simulink model "proc_control_ros2"  (R2024a)
settings: Solver=FixedStepAuto  StartTime=0.0  StopTime=inf  RelTol=1e-3
InitFcn:
  | InitProcControl;
StartFcn:
  | LoadParams;
values from neighbouring files (symbols this model uses):
  A = T200Spec16V{:,3}    [InitProcControl.m]
  dmax = simulation.drift.nominal .* rand(1,6)    [InitProcControl.m]
  dmin = -simulation.drift.nominal .* rand(1,6)    [InitProcControl.m]
  dSeedX = round(rand*10)    [InitProcControl.m]
  dts = 5    [InitProcControl.m]
  N = T200Spec16V{:,6}    [InitProcControl.m]
  PWM = T200Spec16V{:,1}    [InitProcControl.m]
  RPM = T200Spec16V{:,2}    [InitProcControl.m]
undefined symbols (not defined in the file or in its folder): angular_velocity, current_gains, data, data_SL_Info, DiscIntNeverNeededParam, elevation, heading, is_mpc_alive, is_trajectory_done, linear_acceleration, motor1, motor2, motor3, motor4, motor5, motor6, motor7, motor8, MPC, mpc_mode, mpc_status, orientation, physics, pose, position, simulation, simulink, target_reached, thrusters_status, thrusters_status_SL_Info, twist, x_vel_btm, y_vel_btm, z_vel_btm
libraries: ros2lib x79, aerolibutil x12, simulink x9, mpclib x3, embmathops x2, sharedtransform x2, robotcorelib x2, sharedTrackingLibrary x1
(part 1 of 3)
settings Model: SimulationMode=accelerator  PacingRate=1.400000  Creator=relat  LastModifiedBy=nimai
settings OptimizationCC: StrengthReduction=on  PassReuseOutputArgsAs=Individual arguments  ZeroExternalMemoryAtStartup=off  ZeroInternalMemoryAtStartup=off  EfficientFloat2IntCast=on  MaxStackSize=64  OptimizeBlockOrder=speed  MultiThreadedLoops=on  EfficientTunableParamExpr=on
settings DebuggingCC: ParameterTunabilityLossMsg=error
settings HardwareCC: ProdLargestAtomicInteger=Long  ProdLargestAtomicFloat=Double  ProdLongLongMode=on  ProdHWDeviceType=ARM Compatible->ARM 64-bit (LLP64)  TargetBitPerLong=64  TargetBitPerPointer=64  TargetBitPerSizeT=64  TargetBitPerPtrDiffT=64  TargetLargestAtomicFloat=Float  TargetIntDivRoundTo=Zero  TargetEndianess=LittleEndian  TargetWordSize=64  TargetHWDeviceType=AMD->x86-64 (Linux 64)
settings ModelReferenceCC: UpdateModelReferenceTargets=IfOutOfDate  EnableRefExpFcnMdlSchedulingChecks=on  EnableParallelModelReferenceBuilds=on
settings SFSimCC: SFSimEcho=off  MATLABDynamicMemAlloc=off  SimTargetLang=C++
settings RTWCC: Description=Embedded Coder  SystemTargetFile=ert.tlc  HardwareBoard=Robot Operating System 2 (ROS 2)  TLCOptions="-aInlineSetEventsForThisBaseRateFcn=TLC_FALSE -aSuppressMultiTaskScheduler=TLC_FALSE  -aRateBasedStepFcn=0"  GenCodeOnly=on  TemplateMakefile=ert_default_tmf  RetainRTWFile=on  Toolchain=Colcon Tools  BuildConfiguration=Faster Runs  TargetLang=C++
settings CodeAppCC: ForceParamTrailComments=on  IgnoreCustomStorageClasses=off  IgnoreTestpoints=on  OperatorAnnotations=on  SimulinkDataObjDesc=on  SFDataObjDesc=on  InsertBlockDesc=on
settings ERTTargetCC: TargetLangStandard=C++11 (ISO)  UtilityFuncGeneration=Shared location  CodeInterfacePackaging=C++ class  SupportVariableSizeSignals=on  RootIOFormat=Structure reference

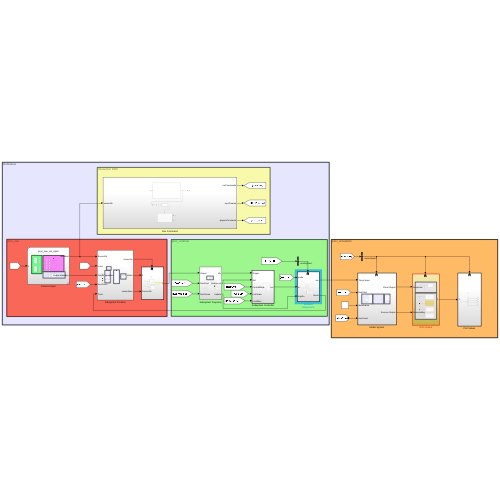
[thumbnail: Simulink's stored preview of the top-level diagram]
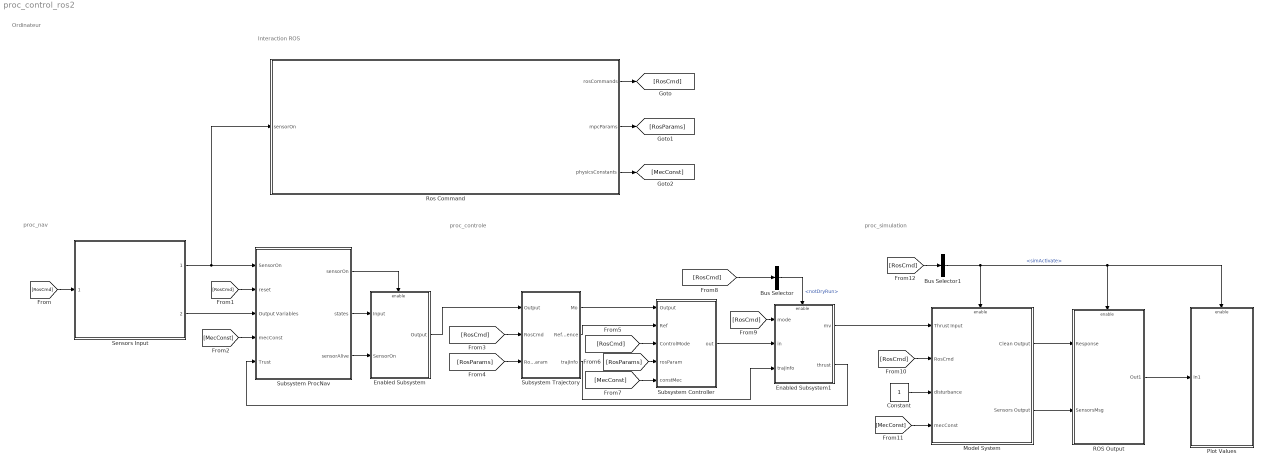
== system proc_control_ros2 ==
  note: Ordinateur
  note: proc_simulation
  note: proc_controle
  note: proc_nav
  note: Interaction ROS
  Bus Selector : BusSelector  OutputSignals=notDryRun
  Bus Selector1 : BusSelector  OutputSignals=simActivate
  Constant : Constant
  Enabled Subsystem : Subsystem  TreatAsAtomicUnit=on
  Enabled Subsystem1 : Subsystem  TreatAsAtomicUnit=on
  Model System : Subsystem  TreatAsAtomicUnit=on
  Plot Values : Subsystem  TreatAsAtomicUnit=on
  ROS Output : Subsystem  TreatAsAtomicUnit=on
  Ros Command : Subsystem
  Sensors Input : Subsystem  ReferencedSubsystem=proc_nav_ros_input
  Subsystem Controller : Subsystem  TreatAsAtomicUnit=on  SystemSampleTime=MPC.Ts
  Subsystem ProcNav : Subsystem
  Subsystem Trajectory : Subsystem
  wires:
  Ros Command/1(rosCommands) -> [RosCmd]
  Ros Command/2(mpcParams) -> [RosParams]
  Ros Command/3(physicsConstants) -> [MecConst]
  [RosCmd] -> Sensors Input/1
  Sensors Input/1 -> Ros Command/1(sensorOn), Subsystem ProcNav/1(SensorOn)
  [RosCmd] -> Subsystem ProcNav/2(reset)
  Sensors Input/2 -> Subsystem ProcNav/3(Output Variables)
  [MecConst] -> Subsystem ProcNav/4(mecConst)
  Subsystem ProcNav/1(sensorOn) -> Enabled Subsystem/Enable
  Subsystem ProcNav/2(states) -> Enabled Subsystem/1(Input)
  Subsystem ProcNav/3(sensorAlive) -> Enabled Subsystem/2(SensorOn)
  Enabled Subsystem/1(Output) -> Subsystem Trajectory/1(Output)
  [RosCmd] -> Subsystem Trajectory/2(RosCmd)
  [RosParams] -> Subsystem Trajectory/3(RosParam)
  Subsystem Trajectory/1(Mo) -> Subsystem Controller/1(Output)
  Subsystem Trajectory/2(Reference) -> Subsystem Controller/2(Ref)
  [RosCmd] -> Subsystem Controller/3(ControlMode)
  [RosParams] -> Subsystem Controller/4(rosParam)
  [MecConst] -> Subsystem Controller/5(constMec)
  Bus Selector/1 -> Enabled Subsystem1/Enable  "<notDryRun>"
  [RosCmd] -> Bus Selector/1
  [RosCmd] -> Enabled Subsystem1/1(mode)
  Subsystem Controller/1(out) -> Enabled Subsystem1/2(in)
  Subsystem Trajectory/3(trajInfo) -> Enabled Subsystem1/3(trajInfo)
  Enabled Subsystem1/2(thrust) -> Subsystem ProcNav/5(Trust)
  Enabled Subsystem1/1(mv) -> Model System/1(Thrust Input)
  [RosCmd] -> Model System/2(RosCmd)
  Constant/1 -> Model System/3(disturbance)
  [MecConst] -> Model System/4(mecConst)
  [RosCmd] -> Bus Selector1/1
  Bus Selector1/1 -> Plot Values/Enable, ROS Output/Enable, Model System/Enable  "<simActivate>"
  Model System/1(Clean Output) -> ROS Output/1(Response)
  Model System/2(Sensors Output) -> ROS Output/2(SensorsMsg)
  ROS Output/1(Out1) -> Plot Values/1(In1)

== system proc_control_ros2/Enabled Subsystem ==
  note: Skipped Commented Blocks
  Input : Inport
  SensorOn : Inport  Port=2
  Enable : EnablePort
  Send Sensor On : Subsystem
  Send auv states : Subsystem
  Output : Outport
  wires:
  Input/1 -> Output/1, Send auv states/1(Input)
  SensorOn/1 -> Send Sensor On/1(IsReached)

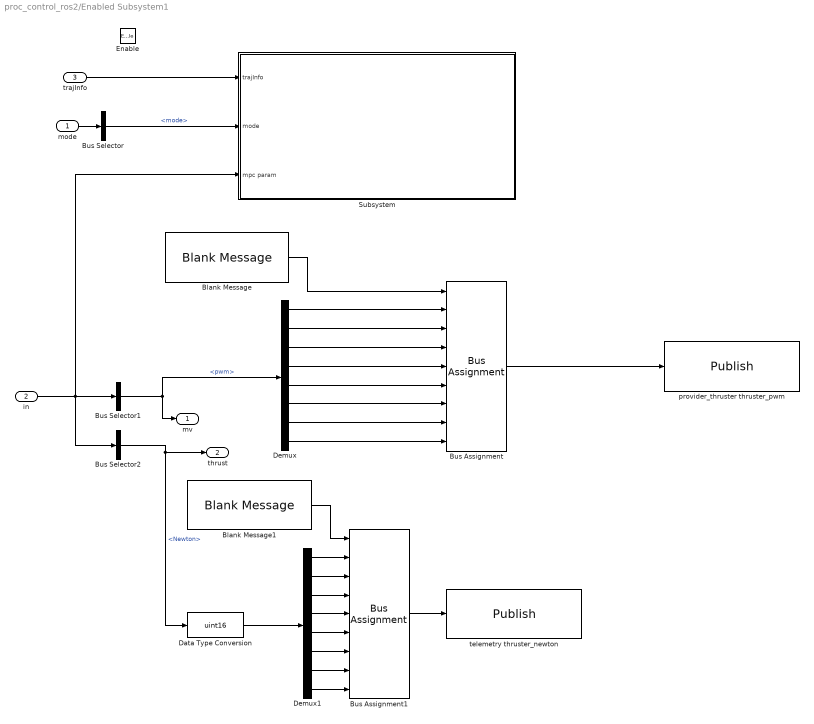
== system proc_control_ros2/Enabled Subsystem1 ==
  mode : Inport
  in : Inport  Port=2
  trajInfo : Inport  Port=3
  Enable : EnablePort
  Blank Message : ros2lib/Blank Message  messageClass=Message  entityType=sonia_common_ros2/MotorPwm  messageType=sonia_common_ros2/MotorPwm  SampleTime=inf
  Blank Message1 : ros2lib/Blank Message  messageClass=Message  entityType=sonia_common_ros2/MotorPwm  messageType=sonia_common_ros2/MotorPwm  SampleTime=inf
  Bus Assignment : BusAssignment  AssignedSignals=motor1,motor2,motor3,motor4,motor5,motor6,motor7,motor8
  Bus Assignment1 : BusAssignment  AssignedSignals=motor1,motor2,motor3,motor4,motor5,motor6,motor7,motor8
  Bus Selector : BusSelector  OutputSignals=mode
  Bus Selector1 : BusSelector  OutputSignals=pwm
  Bus Selector2 : BusSelector  OutputSignals=Newton
  Data Type Conversion : DataTypeConversion  OutDataTypeStr=uint16  SaturateOnIntegerOverflow=off  RndMeth=Floor
  Demux : Demux  Outputs=8
  Demux1 : Demux  Outputs=8
  Subsystem : Subsystem
  provider_thruster thruster_pwm : ros2lib/Publish  topicSource=Specify your own  topic=/provider_thruster/thruster_pwm  messageType=sonia_common_ros2/MotorPwm  QOSHistory=Keep last  QOSDepth=1  QOSReliability=Reliable  QOSDurability=Volatile  QOSDeadline=Inf  QOSLifespan=Inf  QOSLiveliness=Automatic  QOSLeaseDuration=Inf  QOSAvoidROSNamespaceConventions=off
  telemetry thruster_newton : ros2lib/Publish  topicSource=Specify your own  topic=/telemetry/thruster_newton  messageType=sonia_common_ros2/MotorPwm  QOSHistory=Keep last  QOSDepth=1  QOSReliability=Reliable  QOSDurability=Volatile  QOSDeadline=Inf  QOSLifespan=Inf  QOSLiveliness=Automatic  QOSLeaseDuration=Inf  QOSAvoidROSNamespaceConventions=off
  mv : Outport
  thrust : Outport  Port=2
  wires:
  trajInfo/1 -> Subsystem/1(trajInfo)
  mode/1 -> Bus Selector/1
  in/1 -> Subsystem/3(mpc param), Bus Selector2/1, Bus Selector1/1
  Bus Selector1/1 -> Demux/1, mv/1  "<pwm>"
  Bus Selector2/1 -> thrust/1, Data Type Conversion/1  "<Newton>"
  Blank Message/1 -> Bus Assignment/1
  Bus Assignment/1 -> provider_thruster thruster_pwm/1
  Bus Assignment1/1 -> telemetry thruster_newton/1
  Demux1/4 -> Bus Assignment1/5
  Demux1/1 -> Bus Assignment1/2
  Demux1/2 -> Bus Assignment1/3
  Blank Message1/1 -> Bus Assignment1/1
  Demux1/3 -> Bus Assignment1/4
  Demux1/5 -> Bus Assignment1/6
  Demux1/6 -> Bus Assignment1/7
  Demux1/7 -> Bus Assignment1/8
  Demux1/8 -> Bus Assignment1/9
  Data Type Conversion/1 -> Demux1/1
  Bus Selector/1 -> Subsystem/2(mode)  "<mode>"
  Demux/5 -> Bus Assignment/6
  Demux/6 -> Bus Assignment/7
  Demux/7 -> Bus Assignment/8
  Demux/8 -> Bus Assignment/9
  Demux/1 -> Bus Assignment/2
  Demux/2 -> Bus Assignment/3
  Demux/3 -> Bus Assignment/4
  Demux/4 -> Bus Assignment/5

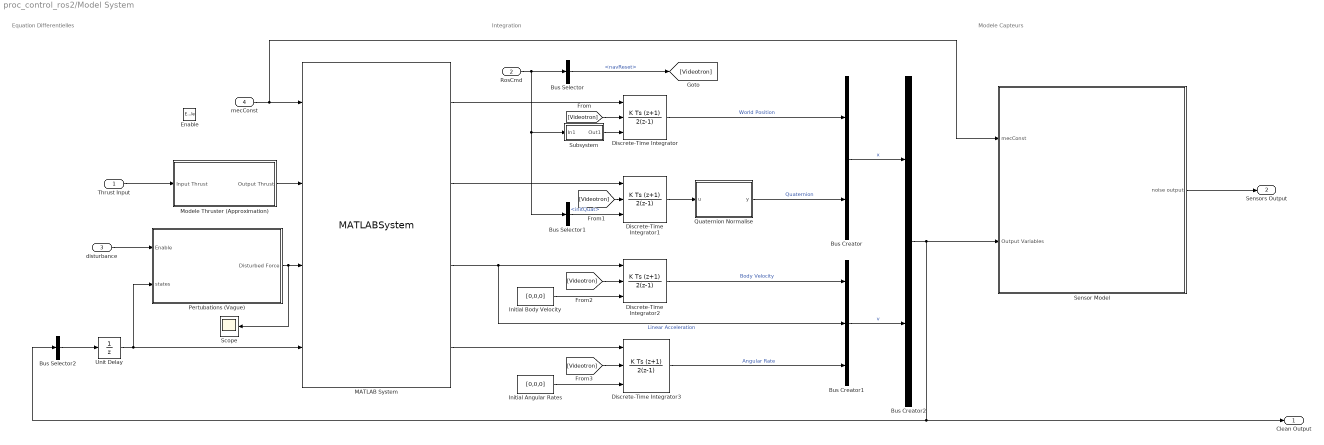
== system proc_control_ros2/Model System ==
  note: Modele Capteurs
  note: Integration
  note: Equation Differentielles
  Thrust Input : Inport
  RosCmd : Inport  Port=2
  disturbance : Inport  Port=3
  mecConst : Inport  Port=4
  Enable : EnablePort
  Bus Creator : BusCreator  Inputs=2
  Bus Creator1 : BusCreator  Inputs=3
  Bus Creator2 : BusCreator  Inputs=2
  Bus Selector : BusSelector  OutputSignals=navReset
  Bus Selector1 : BusSelector  OutputSignals=initQuat
  Bus Selector2 : BusSelector  OutputSignals=x.World Position,x.Quaternion,v.Body Velocity,v.Angular Rate  OutputAsBus=on
  Discrete-Time Integrator{,1..3} (4 alike) : DiscreteIntegrator  IntegratorMethod=Integration: Trapezoidal  ExternalReset=rising  InitialConditionSource=external  SampleTime=simulink.sampletime  ICPrevOutput=DiscIntNeverNeededParam  ICPrevScaledInput=DiscIntNeverNeededParam
  Initial Angular Rates : Constant  Value=[0,0,0]
  Initial Body Velocity : Constant  Value=[0,0,0]
  MATLAB System : MATLABSystem  System=AuvDifferentialEquation  simulation=simulation  MPC=MPC  useDynamicsConst=off  SimulateUsing=Code generation
      mask Type: AuvDifferentialEquation
      mask Display:
      | disp('AuvDifferentialEquation');
      | port_label('input',1,'mecConst');
      | port_label('input',2,'thrust');
      | port_label('input',3,'perturbations');
      | port_label('input',4,'states');
      | port_label('output',1,'Position_dot');
      | port_label('output',2,'Quaternion_dot');
      | port_label('output',3,'BodyVelocity_dot');
      | port_label('output',4,'AngularRates_dot');
  Modele Thruster (Approximation) : Subsystem
  Pertubations (Vague) : Subsystem
  Quaternion Normalise : MATLAB Function  TreatAsAtomicUnit=on
  Scope : Scope
  Sensor Model : Subsystem
  Subsystem : Subsystem
  Unit Delay : UnitDelay  InitialCondition=MPC.Xi  SampleTime=simulink.sampletime  HasFrameUpgradeWarning=on
  Clean Output : Outport
  Sensors Output : Outport  Port=2
  wires:
  Thrust Input/1 -> Modele Thruster (Approximation)/1(Input Thrust)
  disturbance/1 -> Pertubations (Vague)/1(Enable)
  Modele Thruster (Approximation)/1(Output Thrust) -> MATLAB System/2
  Pertubations (Vague)/1(Disturbed Force) -> Scope/1, MATLAB System/3
  mecConst/1 -> Sensor Model/1(mecConst), MATLAB System/1
  RosCmd/1 -> Bus Selector1/1, Subsystem/1(In1), Bus Selector/1
  Bus Selector/1 -> [Videotron]  "<navReset>"
  Subsystem/1(Out1) -> Discrete-Time Integrator/3
  [Videotron] -> Discrete-Time Integrator/2
  MATLAB System/1 -> Discrete-Time Integrator/1
  MATLAB System/2 -> Discrete-Time Integrator1/1
  Bus Selector1/1 -> Discrete-Time Integrator1/3  "<initQuat>"
  [Videotron] -> Discrete-Time Integrator1/2
  Discrete-Time Integrator1/1 -> Quaternion Normalise/1(u)
  [Videotron] -> Discrete-Time Integrator2/2
  Initial Body Velocity/1 -> Discrete-Time Integrator2/3
  Discrete-Time Integrator/1 -> Bus Creator/1  "World Position"
  Quaternion Normalise/1(y) -> Bus Creator/2  "Quaternion"
  MATLAB System/4 -> Discrete-Time Integrator3/1
  Initial Angular Rates/1 -> Discrete-Time Integrator3/3
  [Videotron] -> Discrete-Time Integrator3/2
  Discrete-Time Integrator2/1 -> Bus Creator1/1  "Body Velocity"
  Discrete-Time Integrator3/1 -> Bus Creator1/3  "Angular Rate"
  MATLAB System/3 -> Bus Creator1/2, Discrete-Time Integrator2/1  "Linear Acceleration"
  Bus Creator/1 -> Bus Creator2/1  "x"
  Bus Creator1/1 -> Bus Creator2/2  "v"
  Bus Creator2/1 -> Sensor Model/2(Output Variables), Bus Selector2/1, Clean Output/1
  Bus Selector2/1 -> Unit Delay/1
  Unit Delay/1 -> MATLAB System/4, Pertubations (Vague)/2(states)
  Sensor Model/1(noise output) -> Sensors Output/1

== system proc_control_ros2/Plot Values ==
  In1 : Inport
  Enable : EnablePort
  Bus Selector : BusSelector  OutputSignals=x.World Position,x.Quaternion,v.Body Velocity,v.Angular Rate
  Scope{,1..3} (4 alike) : Scope
  wires:
  In1/1 -> Bus Selector/1
  Bus Selector/1 -> Scope/1  "<World Position>"
  Bus Selector/2 -> Scope1/1  "<Quaternion>"
  Bus Selector/3 -> Scope2/1  "<Body Velocity>"
  Bus Selector/4 -> Scope3/1  "<Angular Rate>"

== system proc_control_ros2/ROS Output ==
  note: Sensor msg
  note: Simulator msg
  Response : Inport
  SensorsMsg : Inport  Port=2
  Enable : EnablePort
  Send DVL msg : Subsystem
  Send Depth msg : Subsystem
  Send IMU Msg : Subsystem
  Send Ping msg : Subsystem  Commented=on
  Send to Unity : Subsystem
  Out1 : Outport
  wires:
  Response/1 -> Send to Unity/1(Response), Out1/1
  SensorsMsg/1 -> Send Ping msg/1(Mesure), Send Depth msg/1(Mesure), Send DVL msg/1(Response), Send IMU Msg/1(Response)

== system proc_control_ros2/Ros Command ==
  sensorOn : Inport
  Bus Selector : BusSelector  OutputSignals=mode
  Get_ROS_param : Subsystem  TreatAsAtomicUnit=on
  If : If  IfExpression=u1 == 0  ShowElse=off
  Ros Command Manager : Subsystem
  Zero-Order Hold : ZeroOrderHold  SampleTime=simulink.ros.paramSampletime
  rosCommands : Outport
  mpcParams : Outport  Port=2
  physicsConstants : Outport  Port=3
  wires:
  Ros Command Manager/1(rosCommands) -> rosCommands/1, Bus Selector/1
  Get_ROS_param/1(mpcParams) -> mpcParams/1
  Zero-Order Hold/1 -> If/1
  Bus Selector/1 -> Zero-Order Hold/1  "<mode>"
  If/1 -> Get_ROS_param/Action
  sensorOn/1 -> Ros Command Manager/1(sensorOn)
  Get_ROS_param/2(physicsConstants) -> physicsConstants/1

== system proc_control_ros2/Subsystem Controller ==
  Output : Inport
  Ref : Inport  Port=2
  ControlMode : Inport  Port=3
  rosParam : Inport  Port=4
  constMec : Inport  Port=5
  Bus Selector : BusSelector  OutputSignals=mode
  Bus Selector1 : BusSelector  OutputSignals=current
  Controller List : Subsystem
  Delay : Delay  DelayLength=1  InitialCondition=zeros(1,8)  SampleTime=MPC.Ts
  If : If  IfExpression=u1 >= 0  ShowElse=off
  If Action Subsystem : Subsystem  TreatAsAtomicUnit=on
  Post Traitement : Subsystem
  out : Outport
  wires:
  Output/1 -> Controller List/1(mo), If Action Subsystem/2(mo)
  ControlMode/1 -> Bus Selector/1
  Bus Selector/1 -> Controller List/2(ControlMode), If Action Subsystem/1(mode), If/1  "<mode>"
  If/1 -> If Action Subsystem/Action
  rosParam/1 -> If Action Subsystem/4(mpcParams)
  If Action Subsystem/1(MPC param) -> Post Traitement/2(MpcParams), Controller List/4(mpc param)
  constMec/1 -> Controller List/5(constMec)
  Ref/1 -> Controller List/3(Ref)
  Controller List/1(Out1) -> Post Traitement/1(In1)
  Post Traitement/1(out) -> Bus Selector1/1, out/1
  Bus Selector1/1 -> Delay/1  "<current>"
  Delay/1 -> If Action Subsystem/3(Current)

== system proc_control_ros2/Subsystem ProcNav ==
  note: Skipped Commented Block
  note: Mettre les données
      | dans un bus
  note: Filtre EKF
  note: Pre traitement des mesures
  note: Conditions pour activer le kalman
  SensorOn : Inport
  reset : Inport  Port=2
  Output Variables : Inport  Port=3
  mecConst : Inport  Port=4
  Trust : Inport  Port=5
  AHRS/Detph Mesurments : Subsystem
  Bus Selector : BusSelector  OutputSignals=navReset
  Bus Selector1 : BusSelector  OutputSignals=NewDvlMsg
  Bus Selector2 : BusSelector  OutputSignals=new Pressure Msg
  DVL Measurements : Subsystem  TreatAsAtomicUnit=on
  Depth Measurements : Subsystem  TreatAsAtomicUnit=on
  Enabled Subsystem : Subsystem  TreatAsAtomicUnit=on
  Reset Logic : Subsystem
  State function arguments : Subsystem
  mux2Bus : Subsystem
  sensorOn : Outport
  states : Outport  Port=2
  sensorAlive : Outport  Port=3
  wires:
  reset/1 -> Bus Selector/1
  Bus Selector/1 -> Reset Logic/1(In1)  "<navReset>"
  SensorOn/1 -> sensorAlive/1, Reset Logic/2(2)
  Reset Logic/1(Out1) -> Enabled Subsystem/Enable, sensorOn/1
  Trust/1 -> State function arguments/1(thrust)
  mecConst/1 -> DVL Measurements/2(mecConst), Enabled Subsystem/5(mecConst), Depth Measurements/2(mecConst), State function arguments/2(mecConst)
  Output Variables/1 -> DVL Measurements/1(DVL Velocity), Bus Selector2/1, Depth Measurements/1(y), Bus Selector1/1, AHRS/Detph Mesurments/1(y)
  Bus Selector1/1 -> DVL Measurements/Enable  "<NewDvlMsg>"
  Bus Selector2/1 -> Depth Measurements/Enable  "<new Pressure Msg>"
  AHRS/Detph Mesurments/1(IMU) -> Depth Measurements/3(xhat), Enabled Subsystem/2(AHRS Mesurments)
  State function arguments/1(stateFuncArguments) -> Enabled Subsystem/1(stateFuncArguments)
  DVL Measurements/1(DVL Measurements) -> Enabled Subsystem/3("DVL Measurements ")
  Depth Measurements/1(Depth Measurements) -> Enabled Subsystem/4(Depth Measurements)
  Enabled Subsystem/1(xhat) -> mux2Bus/1(xhat)
  mux2Bus/1(states) -> states/1  "md"

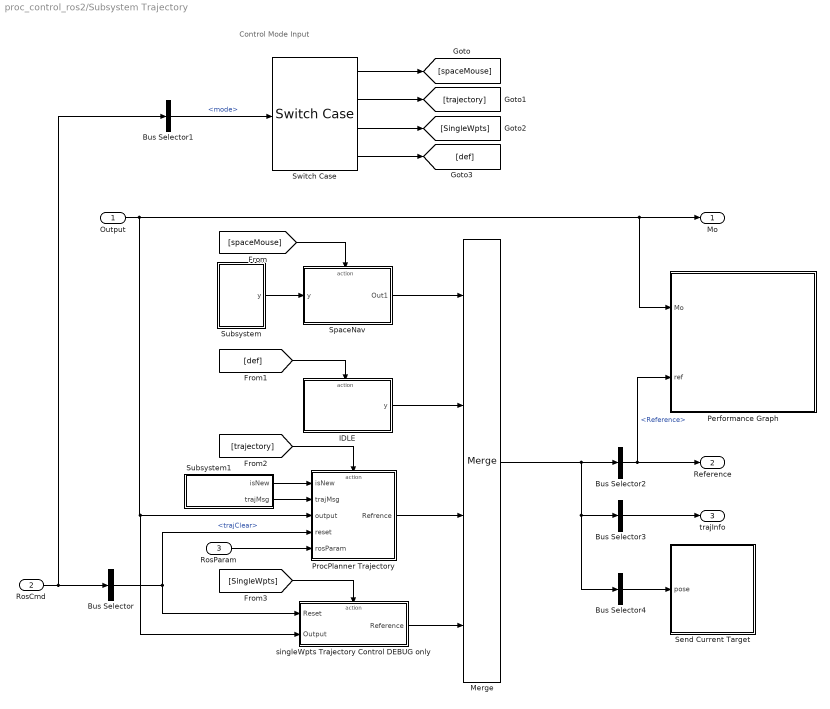
== system proc_control_ros2/Subsystem Trajectory ==
  note: Control Mode Input
  Output : Inport
  RosCmd : Inport  Port=2
  RosParam : Inport  Port=3
  Bus Selector : BusSelector  OutputSignals=trajClear
  Bus Selector1 : BusSelector  OutputSignals=mode
  Bus Selector2 : BusSelector  OutputSignals=Reference
  Bus Selector3 : BusSelector  OutputSignals=isReached,isTrajDone  OutputAsBus=on
  Bus Selector4 : BusSelector  OutputSignals=target  OutputAsBus=on
  IDLE : Subsystem  TreatAsAtomicUnit=on
  Merge : Merge  Inputs=4
  Performance Graph : Subsystem
  ProcPlanner Trajectory : Subsystem  TreatAsAtomicUnit=on
  Send Current Target : Subsystem
  SpaceNav : Subsystem  TreatAsAtomicUnit=on
  Subsystem : Subsystem
  Subsystem1 : Subsystem
  Switch Case : SwitchCase  CaseConditions={mode.traj.SpaceMouseMode,mode.traj.trajMode, mode.traj.singleWpts,}
  singleWpts Trajectory Control DEBUG only : Subsystem  TreatAsAtomicUnit=on
  Mo : Outport
  Reference : Outport  Port=2
  trajInfo : Outport  Port=3
  wires:
  RosCmd/1 -> Bus Selector1/1, Bus Selector/1
  Bus Selector1/1 -> Switch Case/1  "<mode>"
  Switch Case/1 -> [spaceMouse]
  Switch Case/2 -> [trajectory]
  Switch Case/3 -> [SingleWpts]
  Switch Case/4 -> [def]
  Output/1 -> singleWpts Trajectory Control DEBUG only/2(Output), ProcPlanner Trajectory/3(output), Performance Graph/1(Mo), Mo/1
  [spaceMouse] -> SpaceNav/Action
  Subsystem/1(y) -> SpaceNav/1(y)
  [def] -> IDLE/Action
  [trajectory] -> ProcPlanner Trajectory/Action
  Subsystem1/1(isNew) -> ProcPlanner Trajectory/1(isNew)
  Subsystem1/2(trajMsg) -> ProcPlanner Trajectory/2(trajMsg)
  Bus Selector/1 -> singleWpts Trajectory Control DEBUG only/1(Reset), ProcPlanner Trajectory/4(reset)  "<trajClear>"
  RosParam/1 -> ProcPlanner Trajectory/5(rosParam)
  [SingleWpts] -> singleWpts Trajectory Control DEBUG only/Action
  SpaceNav/1(Out1) -> Merge/1
  IDLE/1(y) -> Merge/2
  ProcPlanner Trajectory/1(Refrence) -> Merge/3
  singleWpts Trajectory Control DEBUG only/1(Reference) -> Merge/4
  Merge/1 -> Bus Selector4/1, Bus Selector3/1, Bus Selector2/1
  Bus Selector2/1 -> Performance Graph/2(ref), Reference/1  "<Reference>"
  Bus Selector3/1 -> trajInfo/1
  Bus Selector4/1 -> Send Current Target/1(pose)

== system proc_control_ros2/Enabled Subsystem/Send Sensor On ==
  IsReached : Inport
  Blank Message : ros2lib/Blank Message  messageClass=Message  entityType=std_msgs/Bool  messageType=std_msgs/Bool  SampleTime=inf
  Bus Assignment : BusAssignment  AssignedSignals=data
  Data Type Conversion : DataTypeConversion  OutDataTypeStr=boolean  SaturateOnIntegerOverflow=off  RndMeth=Floor
  Zero-Order Hold : ZeroOrderHold
  proc_control sensor_on : ros2lib/Publish  topicSource=Specify your own  topic=/proc_control/sensor_on  messageType=std_msgs/Bool  QOSHistory=Keep last  QOSDepth=1  QOSReliability=Reliable  QOSDurability=Volatile  QOSDeadline=Inf  QOSLifespan=Inf  QOSLiveliness=Automatic  QOSLeaseDuration=Inf  QOSAvoidROSNamespaceConventions=off
  wires:
  Bus Assignment/1 -> Zero-Order Hold/1
  Zero-Order Hold/1 -> proc_control sensor_on/1
  Data Type Conversion/1 -> Bus Assignment/2
  Blank Message/1 -> Bus Assignment/1
  IsReached/1 -> Data Type Conversion/1

== system proc_control_ros2/Enabled Subsystem/Send auv states ==
  Input : Inport
  Blank Message : ros2lib/Blank Message  messageClass=Message  entityType=nav_msgs/Odometry  messageType=nav_msgs/Odometry  SampleTime=inf
  Bus Assignment : BusAssignment  AssignedSignals=pose.pose.position.x,pose.pose.position.y,pose.pose.position.z,pose.pose.orientation.w,pose.pose.orientation.x,pose.pose.orientation.y,pose.pose.orientation.z,twist.twist.linear.x,twist.twist.linear.y,twist.twist.linear.z,twist.twist.angular.x,twist.twist.angular.y,twist.twist.angular.z
  Demux : Demux  Outputs=13
  Header Assignment : ros2lib/Header Assignment  SetFrameID=on  FrameID=NED  InsertTimeStamp=on  SetHeaderFieldName=Use the default header field name  HeaderFieldName=header
  bus2mux : Subsystem
  proc_nav auv_states : ros2lib/Publish  topicSource=Specify your own  topic=/proc_nav/auv_states  messageType=nav_msgs/Odometry  QOSHistory=Keep last  QOSDepth=1  QOSReliability=Reliable  QOSDurability=Volatile  QOSDeadline=Inf  QOSLifespan=5  QOSLiveliness=Automatic  QOSLeaseDuration=5  QOSAvoidROSNamespaceConventions=off
  wires:
  Blank Message/1 -> Header Assignment/1
  Input/1 -> bus2mux/1(Input)
  Header Assignment/1 -> Bus Assignment/1
  bus2mux/1(states) -> Demux/1
  Demux/1 -> Bus Assignment/2
  Demux/2 -> Bus Assignment/3
  Demux/3 -> Bus Assignment/4
  Demux/4 -> Bus Assignment/5
  Demux/5 -> Bus Assignment/6
  Demux/6 -> Bus Assignment/7
  Demux/7 -> Bus Assignment/8
  Demux/8 -> Bus Assignment/9
  Demux/9 -> Bus Assignment/10
  Demux/10 -> Bus Assignment/11
  Demux/11 -> Bus Assignment/12
  Demux/12 -> Bus Assignment/13
  Demux/13 -> Bus Assignment/14
  Bus Assignment/1 -> proc_nav auv_states/1

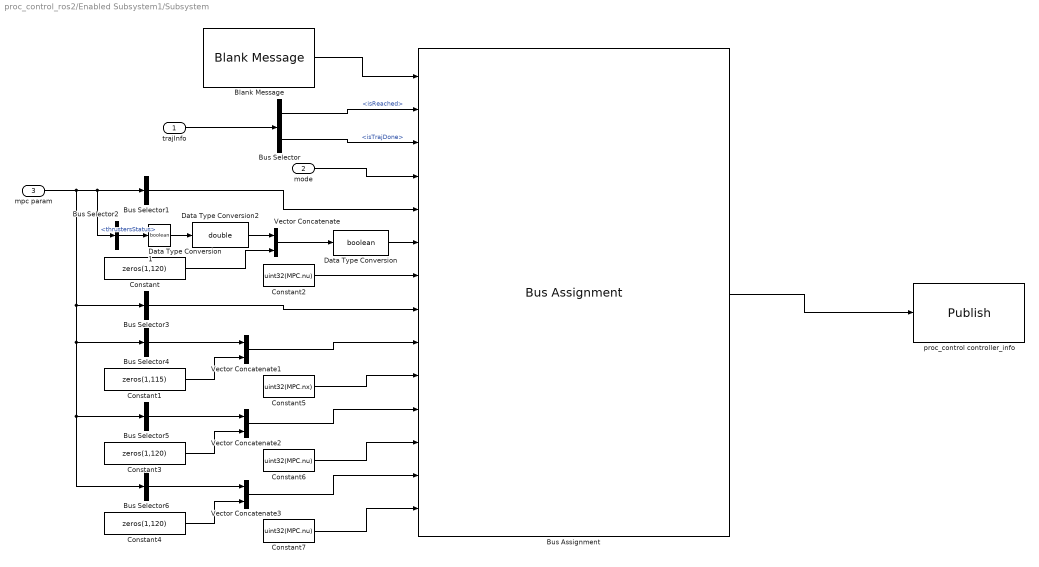
== system proc_control_ros2/Enabled Subsystem1/Subsystem ==
  trajInfo : Inport
  mode : Inport  Port=2
  mpc param : Inport  Port=3  SampleTime=0.02
  Blank Message : ros2lib/Blank Message  messageClass=Message  entityType=sonia_common_ros2/MpcInfo  messageType=sonia_common_ros2/MpcInfo  SampleTime=inf
  Bus Assignment : BusAssignment  AssignedSignals=target_reached,is_trajectory_done,mpc_mode,is_mpc_alive,thrusters_status,thrusters_status_SL_Info.CurrentLength,mpc_status,current_gains.ov,current_gains.ov_SL_Info.CurrentLength,current_gains.mv,current_gains.mv_SL_Info.CurrentLength,current_gains.mvr,current_gains.mvr_SL_Info.CurrentLength
  Bus Selector : BusSelector  OutputSignals=isReached,isTrajDone
  Bus Selector1 : BusSelector  OutputSignals=isMpcAlive  OutputAsBus=on
  Bus Selector2 : BusSelector  OutputSignals=mpcParams.thrustersStatus
  Bus Selector3 : BusSelector  OutputSignals=MpcStatus  OutputAsBus=on
  Bus Selector4 : BusSelector  OutputSignals=mpcParams.ywt  OutputAsBus=on
  Bus Selector5 : BusSelector  OutputSignals=mpcParams.mvwt  OutputAsBus=on
  Bus Selector6 : BusSelector  OutputSignals=mpcParams.dmwwt  OutputAsBus=on
  Constant : Constant  Value=zeros(1,120)  VectorParams1D=off
  Constant1 : Constant  Value=zeros(1,115)  VectorParams1D=off
  Constant2 : Constant  Value=uint32(MPC.nu)
  Constant3 : Constant  Value=zeros(1,120)  VectorParams1D=off
  Constant4 : Constant  Value=zeros(1,120)  VectorParams1D=off
  Constant5 : Constant  Value=uint32(MPC.nx)  VectorParams1D=off
  Constant6 : Constant  Value=uint32(MPC.nu)
  Constant7 : Constant  Value=uint32(MPC.nu)
  Data Type Conversion : DataTypeConversion  OutDataTypeStr=boolean  SaturateOnIntegerOverflow=off  RndMeth=Floor
  Data Type Conversion1 : DataTypeConversion  OutDataTypeStr=boolean  SaturateOnIntegerOverflow=off  RndMeth=Floor
  Data Type Conversion2 : DataTypeConversion  OutDataTypeStr=double  SaturateOnIntegerOverflow=off  RndMeth=Floor
  Vector Concatenate{,1..3} (4 alike) : Concatenate
  proc_control controller_info : ros2lib/Publish  topicSource=Specify your own  topic=proc_control/controller_info  messageType=sonia_common_ros2/MpcInfo  QOSHistory=Keep last  QOSDepth=1  QOSReliability=Reliable  QOSDurability=Volatile  QOSDeadline=Inf  QOSLifespan=Inf  QOSLiveliness=Automatic  QOSLeaseDuration=Inf  QOSAvoidROSNamespaceConventions=off
  wires:
  Constant7/1 -> Bus Assignment/14
  Vector Concatenate3/1 -> Bus Assignment/13
  Constant6/1 -> Bus Assignment/12
  Vector Concatenate2/1 -> Bus Assignment/11
  Constant5/1 -> Bus Assignment/10
  Vector Concatenate1/1 -> Bus Assignment/9
  Constant2/1 -> Bus Assignment/7
  Vector Concatenate/1 -> Data Type Conversion/1
  Bus Selector/2 -> Bus Assignment/3  "<isTrajDone>"
  mpc param/1 -> Bus Selector6/1, Bus Selector5/1, Bus Selector4/1, Bus Selector3/1, Bus Selector2/1, Bus Selector1/1
  mode/1 -> Bus Assignment/4
  trajInfo/1 -> Bus Selector/1
  Constant3/1 -> Vector Concatenate2/2
  Bus Selector4/1 -> Vector Concatenate1/1
  Bus Selector2/1 -> Data Type Conversion1/1  "<thrustersStatus>"
  Bus Selector6/1 -> Vector Concatenate3/1
  Constant/1 -> Vector Concatenate/2
  Bus Selector3/1 -> Bus Assignment/8
  Bus Selector1/1 -> Bus Assignment/5
  Constant1/1 -> Vector Concatenate1/2
  Bus Selector/1 -> Bus Assignment/2  "<isReached>"
  Bus Selector5/1 -> Vector Concatenate2/1
  Constant4/1 -> Vector Concatenate3/2
  Blank Message/1 -> Bus Assignment/1
  Data Type Conversion/1 -> Bus Assignment/6
  Data Type Conversion1/1 -> Data Type Conversion2/1
  Data Type Conversion2/1 -> Vector Concatenate/1
  Bus Assignment/1 -> proc_control controller_info/1

== system proc_control_ros2/Model System/Modele Thruster (Approximation) ==
  Input Thrust : Inport
  Demux : Demux  Outputs=8
  MATLAB Function : MATLAB Function  TreatAsAtomicUnit=on
  Mux : Mux  Inputs=8
  PWN to N : Lookup_n-D  NumberOfTableDimensions=1  BreakpointsForDimension1=PWM  BreakpointsForDimension3=[5, 7]  BreakpointsForDimension1DataTypeStr=uint16  Table=N  TableDataTypeStr=double  InterpMethod=Nearest  InternalRulePriority=Speed  OutDataTypeStr=double  RndMeth=Simplest
  Send RPM to unity : Subsystem
  T1 : Subsystem
  T2 : Subsystem
  T3 : Subsystem
  T4 : Subsystem
  T5 : Subsystem
  T6 : Subsystem
  T7 : Subsystem
  T8 : Subsystem
  Output Thrust : Outport
  wires:
  Input Thrust/1 -> MATLAB Function/1(u)
  MATLAB Function/1(y) -> PWN to N/1
  PWN to N/1 -> Demux/1
  Demux/1 -> T1/1(In1)
  Demux/2 -> T2/1(In1)
  Demux/3 -> T3/1(In1)
  Demux/4 -> T4/1(In1)
  Demux/5 -> T5/1(In1)
  Demux/8 -> T8/1(In1)
  Demux/6 -> T6/1(In1)
  Demux/7 -> T7/1(In1)
  T1/1(Out1) -> Mux/1
  T2/1(Out1) -> Mux/2
  T3/1(Out1) -> Mux/3
  T4/1(Out1) -> Mux/4
  T5/1(Out1) -> Mux/5
  T6/1(Out1) -> Mux/6
  T7/1(Out1) -> Mux/7
  T8/1(Out1) -> Mux/8
  Mux/1 -> Send RPM to unity/1(In1), Output Thrust/1

== system proc_control_ros2/Model System/Pertubations (Vague) ==
  note: Drift
  note: Wave
  Enable : Inport
  states : Inport  Port=2
  Constant : Constant  Value=simulation.wave.damp.A
  Constant1 : Constant  Value=simulation.wave.damp.B
  Constant2 : Constant  Value=zeros(1,6)
  Drift : UniformRandomNumber  Minimum=dmin  Maximum=dmax  Seed=dSeedX  SampleTime=dts
  Product : Product
  Product1 : Product
  Saturation : Saturate  UpperLimit=simulation.wave.damp.min  LowerLimit=simulation.wave.damp.max
  Selector : Selector  InputPortWidth=13  IndexOptions=Index vector (dialog)  Indices=[3]  OutputSizes=1
  Sine Wave : Sin  SineType=Sample based  Amplitude=simulation.wave.amplitudes  Samples=waveDiscreteFrequency  SampleTime=simulink.sampletime  Offset=waveDiscretePhase
  Sum : Sum  Inputs=|++
  Sum1 : Sum  Inputs=++|
  Switch : Switch  Criteria=u2 > Threshold  SaturateOnIntegerOverflow=off  InputSameDT=off
  Disturbed Force : Outport
  wires:
  Drift/1 -> Sum1/1
  Constant/1 -> Product/2
  states/1 -> Selector/1
  Sum/1 -> Saturation/1
  Selector/1 -> Product/1
  Product/1 -> Sum/1
  Constant1/1 -> Sum/2
  Sine Wave/1 -> Product1/1
  Saturation/1 -> Product1/2
  Switch/1 -> Disturbed Force/1
  Enable/1 -> Switch/2
  Constant2/1 -> Switch/3
  Sum1/1 -> Switch/1
  Product1/1 -> Sum1/2

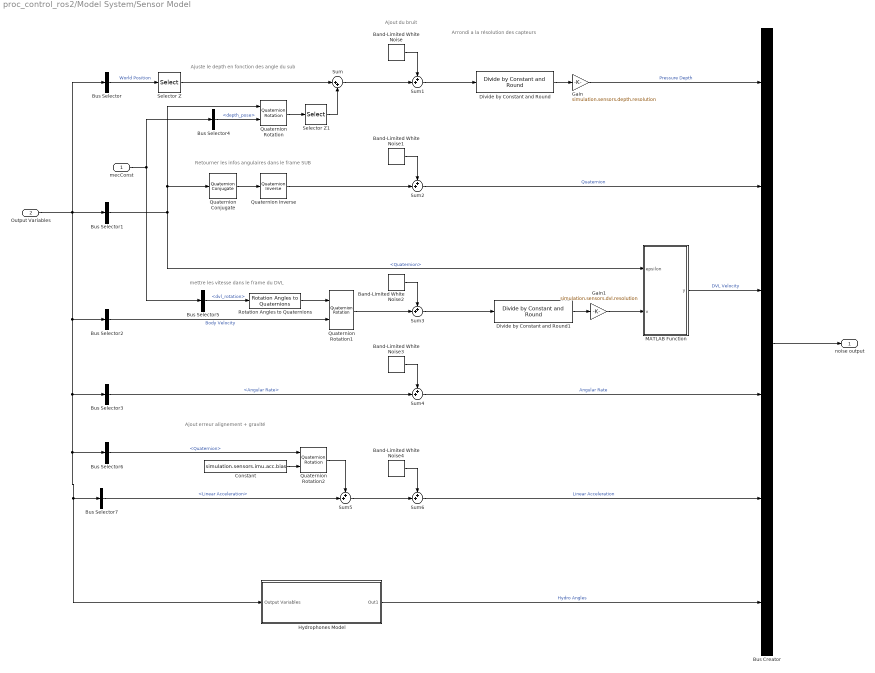
== system proc_control_ros2/Model System/Sensor Model ==
  note: Arrondi a la résolution des capteurs
  note: Ajout du bruit
  note: Ajout erreur alignement + gravité
  note: mettre les vitesse dans le frame du DVL
  note: Retourner les infos angulaires dans le frame SUB
  note: Ajuste le depth en fonction des angle du sub
  mecConst : Inport
  Output Variables : Inport  Port=2
  Band-Limited White Noise{,1..4} (5 alike) : simulink/Sources/Band-Limited White Noise  Cov=[simulation.sensors.noise.power]  Ts=simulation.sensors.noise.sampletime  seed=[23341]
  Bus Creator : BusCreator  Inputs=6
  Bus Selector : BusSelector  OutputSignals=x.World Position  OutputAsBus=on
  Bus Selector1 : BusSelector  OutputSignals=x.Quaternion
  Bus Selector2 : BusSelector  OutputSignals=v.Body Velocity  OutputAsBus=on
  Bus Selector3 : BusSelector  OutputSignals=v.Angular Rate
  Bus Selector4 : BusSelector  OutputSignals=depth_pose
  Bus Selector5 : BusSelector  OutputSignals=dvl_rotation
  Bus Selector6 : BusSelector  OutputSignals=x.Quaternion
  Bus Selector7 : BusSelector  OutputSignals=v.Linear Acceleration
  Constant : Constant  Value=simulation.sensors.imu.acc.bias
  Divide by Constant and Round : embmathops/Divide by Constant and Round  Denominator=simulation.sensors.depth.resolution  RoundingMethod=Nearest  SimulateUsing=Code generation
      settings: LibrarySourceBlock=embeddedMathLib/Divide by Constant and Round
  Divide by Constant and Round1 : embmathops/Divide by Constant and Round  Denominator=simulation.sensors.dvl.resolution  RoundingMethod=Nearest  SimulateUsing=Code generation
      settings: LibrarySourceBlock=embeddedMathLib/Divide by Constant and Round
  Gain : Gain  Gain=simulation.sensors.depth.resolution
  Gain1 : Gain  Gain=simulation.sensors.dvl.resolution
  Hydrophones Model : Subsystem
  MATLAB Function : MATLAB Function  TreatAsAtomicUnit=on
  Quaternion Conjugate : aerolibutil/Quaternion Conjugate
  Quaternion Inverse : aerolibutil/Quaternion Inverse
  Quaternion Rotation : aerolibutil/Quaternion Rotation
  Quaternion Rotation1 : aerolibutil/Quaternion Rotation
  Quaternion Rotation2 : aerolibutil/Quaternion Rotation
  Rotation Angles to Quaternions : sharedtransform/Rotation Angles to Quaternions  rotationOrder=XYZ  aMode=aMode
  Selector Z : Selector  InputPortWidth=3  IndexOptions=Index vector (dialog)  Indices=[3]  OutputSizes=1
  Selector Z1 : Selector  InputPortWidth=3  IndexOptions=Index vector (dialog)  Indices=[3]  OutputSizes=1
  Sum : Sum  Inputs=|++
  Sum{1..6} (6 alike) : Sum  Inputs=++|
  noise output : Outport
  wires:
  Bus Selector/1 -> Selector Z/1  "World Position"
  Bus Selector1/1 -> Quaternion Conjugate/1, Quaternion Rotation/1, MATLAB Function/1(epsilon)  "<Quaternion>"
  Bus Selector2/1 -> Quaternion Rotation1/2  "Body Velocity"
  Bus Selector3/1 -> Sum4/2  "<Angular Rate>"
  Selector Z/1 -> Sum/1
  mecConst/1 -> Bus Selector5/1, Bus Selector4/1
  Bus Selector4/1 -> Quaternion Rotation/2  "<depth_pose>"
  Quaternion Rotation/1 -> Selector Z1/1
  Selector Z1/1 -> Sum/2
  Quaternion Conjugate/1 -> Quaternion Inverse/1
  Bus Selector5/1 -> Rotation Angles to Quaternions/1  "<dvl_rotation>"
  Rotation Angles to Quaternions/1 -> Quaternion Rotation1/1
  Band-Limited White Noise/1 -> Sum1/1
  Sum/1 -> Sum1/2
  Quaternion Inverse/1 -> Sum2/2
  Band-Limited White Noise1/1 -> Sum2/1
  Band-Limited White Noise2/1 -> Sum3/1
  Quaternion Rotation1/1 -> Sum3/2
  Band-Limited White Noise3/1 -> Sum4/1
  Constant/1 -> Quaternion Rotation2/2
  Bus Selector6/1 -> Quaternion Rotation2/1  "<Quaternion>"
  Output Variables/1 -> Hydrophones Model/1(Output Variables), Bus Selector7/1, Bus Selector6/1, Bus Selector3/1, Bus Selector2/1, Bus Selector1/1, Bus Selector/1
  Quaternion Rotation2/1 -> Sum5/1
  Bus Selector7/1 -> Sum5/2  "<Linear Acceleration>"
  Band-Limited White Noise4/1 -> Sum6/1
  Sum5/1 -> Sum6/2
  Sum1/1 -> Divide by Constant and Round/1
  Divide by Constant and Round/1 -> Gain/1
  Sum3/1 -> Divide by Constant and Round1/1
  Divide by Constant and Round1/1 -> Gain1/1
  Gain1/1 -> MATLAB Function/2(v)
  Gain/1 -> Bus Creator/1  "Pressure Depth"
  Sum2/1 -> Bus Creator/2  "Quaternion"
  MATLAB Function/1(y) -> Bus Creator/3  "DVL Velocity"
  Sum4/1 -> Bus Creator/4  "Angular Rate"
  Sum6/1 -> Bus Creator/5  "Linear Acceleration"
  Hydrophones Model/1(Out1) -> Bus Creator/6  "Hydro Angles"
  Bus Creator/1 -> noise output/1

== system proc_control_ros2/Model System/Subsystem ==
  In1 : Inport
  Bus Selector : BusSelector  OutputSignals=initPos
  Constant : Constant  Value=[0,0]
  Mux : Mux  Inputs=2
  Selector : Selector  InputPortWidth=3  IndexOptions=Index vector (dialog)  Indices=[3]  OutputSizes=1
  Out1 : Outport
  wires:
  In1/1 -> Bus Selector/1
  Bus Selector/1 -> Selector/1  "<initPos>"
  Selector/1 -> Mux/2
  Constant/1 -> Mux/1
  Mux/1 -> Out1/1

== system proc_control_ros2/ROS Output/Send DVL msg ==
  Response : Inport
  Blank Message : ros2lib/Blank Message  messageClass=Message  entityType=sonia_common_ros2/BodyVelocityDVL  messageType=sonia_common_ros2/BodyVelocityDVL  SampleTime=inf
  Bus Assignment : BusAssignment  AssignedSignals=x_vel_btm,y_vel_btm,z_vel_btm
  Bus Selector : BusSelector  OutputSignals=DVL Velocity
  Demux : Demux  Outputs=3
  Publish : ros2lib/Publish  topicSource=Specify your own  topic=/proc_simulation/dvl_velocity  messageType=sonia_common_ros2/BodyVelocityDVL  QOSHistory=Keep last  QOSDepth=1  QOSReliability=Reliable  QOSDurability=Volatile  QOSDeadline=Inf  QOSLifespan=Inf  QOSLiveliness=Automatic  QOSLeaseDuration=Inf  QOSAvoidROSNamespaceConventions=off
  wires:
  Demux/3 -> Bus Assignment/4
  Response/1 -> Bus Selector/1
  Bus Selector/1 -> Demux/1  "<DVL Velocity>"
  Blank Message/1 -> Bus Assignment/1
  Bus Assignment/1 -> Publish/1
  Demux/1 -> Bus Assignment/2
  Demux/2 -> Bus Assignment/3

== system proc_control_ros2/ROS Output/Send Depth msg ==
  Mesure : Inport
  Blank Message : ros2lib/Blank Message  messageClass=Message  entityType=std_msgs/Float32  messageType=std_msgs/Float32  SampleTime=inf
  Bus Assignment : BusAssignment  AssignedSignals=data
  Bus Selector : BusSelector  OutputSignals=Pressure Depth
  Data Type Conversion : DataTypeConversion  OutDataTypeStr=single  SaturateOnIntegerOverflow=off  RndMeth=Floor
  Publish : ros2lib/Publish  topicSource=Specify your own  topic=/proc_simulation/depth  messageType=std_msgs/Float32  QOSHistory=Keep last  QOSDepth=1  QOSReliability=Reliable  QOSDurability=Volatile  QOSDeadline=Inf  QOSLifespan=Inf  QOSLiveliness=Automatic  QOSLeaseDuration=Inf  QOSAvoidROSNamespaceConventions=off
  Zero-Order Hold : ZeroOrderHold  SampleTime=simulation.sensors.depth.sampletime
  wires:
  Data Type Conversion/1 -> Bus Assignment/2
  Mesure/1 -> Bus Selector/1
  Zero-Order Hold/1 -> Data Type Conversion/1
  Bus Selector/1 -> Zero-Order Hold/1  "<Pressure Depth>"
  Blank Message/1 -> Bus Assignment/1
  Bus Assignment/1 -> Publish/1

== system proc_control_ros2/ROS Output/Send IMU Msg ==
  Response : Inport
  Blank Message : ros2lib/Blank Message  messageClass=Message  entityType=sensor_msgs/Imu  messageType=sensor_msgs/Imu  SampleTime=inf
  Bus Assignment : BusAssignment  AssignedSignals=angular_velocity.x,angular_velocity.y,angular_velocity.z,orientation.w,orientation.x,orientation.y,orientation.z,linear_acceleration.x,linear_acceleration.y,linear_acceleration.z
  Bus Selector : BusSelector  OutputSignals=Angular Rate,Linear Acceleration,Quaternion
  Demux : Demux  Outputs=3
  Demux1 : Demux
  Demux2 : Demux  Outputs=3
  Header Assignment : ros2lib/Header Assignment  SetFrameID=on  FrameID=NED  InsertTimeStamp=on  SetHeaderFieldName=Use the default header field name  HeaderFieldName=header
  Publish : ros2lib/Publish  topicSource=Specify your own  topic=/proc_simulation/imu_info  messageType=sensor_msgs/Imu  QOSHistory=Keep last  QOSDepth=1  QOSReliability=Reliable  QOSDurability=Volatile  QOSDeadline=Inf  QOSLifespan=Inf  QOSLiveliness=Automatic  QOSLeaseDuration=Inf  QOSAvoidROSNamespaceConventions=off
  wires:
  Blank Message/1 -> Header Assignment/1
  Header Assignment/1 -> Bus Assignment/1
  Response/1 -> Bus Selector/1
  Bus Selector/1 -> Demux/1  "<Angular Rate>"
  Demux/1 -> Bus Assignment/2
  Demux/2 -> Bus Assignment/3
  Demux/3 -> Bus Assignment/4
  Demux1/1 -> Bus Assignment/5
  Demux1/2 -> Bus Assignment/6
  Demux1/3 -> Bus Assignment/7
  Demux1/4 -> Bus Assignment/8
  Bus Selector/3 -> Demux1/1  "<Quaternion>"
  Bus Selector/2 -> Demux2/1  "<Linear Acceleration>"
  Bus Assignment/1 -> Publish/1
  Demux2/1 -> Bus Assignment/9
  Demux2/2 -> Bus Assignment/10
  Demux2/3 -> Bus Assignment/11

== system proc_control_ros2/ROS Output/Send Ping msg ==
  Mesure : Inport
  Blank Message : ros2lib/Blank Message  messageClass=Message  entityType=sonia_common_ros2/PingAngles  messageType=sonia_common_ros2/PingAngles  SampleTime=inf
  Bus Assignment : BusAssignment  AssignedSignals=heading,elevation
  Bus Selector : BusSelector  OutputSignals=Hydro Angles
  Demux : Demux  Outputs=3
  Publish : ros2lib/Publish  topicSource=Specify your own  topic=/proc_simulation/ping  messageType=sonia_common_ros2/PingAngles  QOSHistory=Keep last  QOSDepth=1  QOSReliability=Reliable  QOSDurability=Volatile  QOSDeadline=Inf  QOSLifespan=Inf  QOSLiveliness=Automatic  QOSLeaseDuration=Inf  QOSAvoidROSNamespaceConventions=off
  Terminator : Terminator
  Zero-Order Hold : ZeroOrderHold  SampleTime=simulation.sensors.depth.sampletime
  wires:
  Blank Message/1 -> Bus Assignment/1
  Mesure/1 -> Bus Selector/1
  Bus Selector/1 -> Zero-Order Hold/1  "<Hydro Angles>"
  Demux/1 -> Bus Assignment/2
  Demux/2 -> Bus Assignment/3
  Zero-Order Hold/1 -> Demux/1
  Demux/3 -> Terminator/1
  Bus Assignment/1 -> Publish/1

== system proc_control_ros2/ROS Output/Send to Unity ==
  Response : Inport
  Blank Message : ros2lib/Blank Message  messageClass=Message  entityType=geometry_msgs/Pose  messageType=geometry_msgs/Pose  SampleTime=inf
  Bus Assignment : BusAssignment  AssignedSignals=position.x,position.y,position.z,orientation.x,orientation.y,orientation.z,orientation.w
  Bus Selector : BusSelector  OutputSignals=x.World Position,x.Quaternion
  Demux : Demux  Outputs=3
  Demux1 : Demux
  Publish : ros2lib/Publish  topicSource=Specify your own  topic=proc_simulation/true_states  messageType=geometry_msgs/Pose  QOSHistory=Keep last  QOSDepth=1  QOSReliability=Reliable  QOSDurability=Volatile  QOSDeadline=Inf  QOSLifespan=Inf  QOSLiveliness=Automatic  QOSLeaseDuration=Inf  QOSAvoidROSNamespaceConventions=off
  wires:
  Bus Selector/2 -> Demux1/1  "<Quaternion>"
  Response/1 -> Bus Selector/1
  Bus Selector/1 -> Demux/1  "<World Position>"
  Blank Message/1 -> Bus Assignment/1
  Demux/1 -> Bus Assignment/2
  Demux/2 -> Bus Assignment/3
  Demux/3 -> Bus Assignment/4
  Demux1/1 -> Bus Assignment/5
  Demux1/2 -> Bus Assignment/6
  Demux1/3 -> Bus Assignment/7
  Demux1/4 -> Bus Assignment/8
  Bus Assignment/1 -> Publish/1

== system proc_control_ros2/Ros Command/Get_ROS_param ==
  Action Port : ActionPort  InitializeStates=reset  ActionPortLabel=if(u1 == 0)
  MPC Parameters : Subsystem
  Physics Constants : Subsystem
  mpcParams : Outport
  physicsConstants : Outport  Port=2
  wires:
  Physics Constants/1(physicsConstants) -> physicsConstants/1
  MPC Parameters/1(mpcParams) -> mpcParams/1

== system proc_control_ros2/Ros Command/Ros Command Manager ==
  note: CUSTOM MESSAGE
  sensorOn : Inport
  Bus Creator : BusCreator  Inputs=7
  Bus Selector : BusSelector  OutputSignals=data  OutputAsBus=on
  Bus Selector1 : BusSelector  OutputSignals=data  OutputAsBus=on
  Bus Selector2 : BusSelector  OutputSignals=status  OutputAsBus=on
  Bus Selector3 : BusSelector  OutputSignals=position,orientation  OutputAsBus=on
  Bus Selector4 : BusSelector  OutputSignals=data  OutputAsBus=on
  Data Type Conversion : DataTypeConversion  OutDataTypeStr=uint8  SaturateOnIntegerOverflow=off  RndMeth=Floor
  Delay : Delay  DelayLength=1  InitialCondition=0
  MATLAB System : MATLABSystem  System=rosCommandManager  initial_mode=mode.init  SimulateUsing=Code generation
      mask Type: rosCommandManager
      mask Display:
      | disp('rosCommandManager');
      | port_label('input',1,'newSetMode');
      | port_label('input',2,'setMode');
      | port_label('input',3,'newReset');
      | port_label('input',4,'reset');
      | port_label('input',5,'newKill');
      | port_label('input',6,'kill');
      | port_label('input',7,'newIc');
      | port_label('input',8,'ic');
      | port_label('input',9,'newDryRun');
      | port_label('input',10,'Dryrun');
      | port_label('input',11,'newTrajreset');
      | port_label('input',12,'sensorOn');
      | port_label('output',1,'initQuat');
      | port_label('output',2,'initPos');
      | port_label('output',3,'simEnable');
      | port_label('output',4,'reset');
      | port_label('output',5,'mode');
      | port_label('output',6,'trajClear');
      | port_label('output',7,'notDryRun');
  Terminator : Terminator
  proc_control reset_trajectory : ros2lib/Subscribe  topicSource=Specify your own  topic=/proc_control/reset_trajectory  messageType=std_msgs/Bool  sampleTime=MPC.Ts  QOSHistory=Keep last  QOSDepth=10  QOSReliability=Reliable  QOSDurability=Volatile  QOSDeadline=inf  QOSLifespan=inf  QOSLiveliness=Automatic  QOSLeaseDuration=inf  QOSAvoidROSNamespaceConventions=off
  proc_control set_mode : ros2lib/Subscribe  topicSource=Specify your own  topic=/proc_control/set_mode  messageType=std_msgs/UInt8  sampleTime=MPC.Ts  QOSHistory=Keep last  QOSDepth=10  QOSReliability=Reliable  QOSDurability=Volatile  QOSDeadline=inf  QOSLifespan=inf  QOSLiveliness=Automatic  QOSLeaseDuration=inf  QOSAvoidROSNamespaceConventions=off
  proc_nav reset_pos : ros2lib/Subscribe  topicSource=Specify your own  topic=/proc_nav/reset_pos  messageType=std_msgs/Bool  sampleTime=MPC.Ts  QOSHistory=Keep last  QOSDepth=1  QOSReliability=Reliable  QOSDurability=Volatile  QOSDeadline=Inf  QOSLifespan=Inf  QOSLiveliness=Automatic  QOSLeaseDuration=Inf  QOSAvoidROSNamespaceConventions=off
  proc_simulation start_simulation : ros2lib/Subscribe  topicSource=Specify your own  topic=/proc_simulation/start_simulation  messageType=geometry_msgs/Pose  sampleTime=MPC.Ts  QOSHistory=Keep last  QOSDepth=10  QOSReliability=Reliable  QOSDurability=Volatile  QOSDeadline=inf  QOSLifespan=inf  QOSLiveliness=Automatic  QOSLeaseDuration=inf  QOSAvoidROSNamespaceConventions=off
  provider_rs485 kill_status : ros2lib/Subscribe  topicSource=Specify your own  topic=/provider_rs485/kill_status  messageType=sonia_common_ros2/KillStatus  sampleTime=MPC.Ts  QOSHistory=Keep last  QOSDepth=10  QOSReliability=Reliable  QOSDurability=Volatile  QOSDeadline=inf  QOSLifespan=inf  QOSLiveliness=Automatic  QOSLeaseDuration=inf  QOSAvoidROSNamespaceConventions=off
  telemetry dryrun : ros2lib/Subscribe  topicSource=Specify your own  topic=/telemetry/dry_run  messageType=std_msgs/Bool  sampleTime=MPC.Ts  QOSHistory=Keep last  QOSDepth=10  QOSReliability=Reliable  QOSDurability=Volatile  QOSDeadline=inf  QOSLifespan=inf  QOSLiveliness=Automatic  QOSLeaseDuration=inf  QOSAvoidROSNamespaceConventions=off
  rosCommands : Outport
  wires:
  Bus Selector1/1 -> MATLAB System/4
  Bus Selector4/1 -> MATLAB System/10
  MATLAB System/6 -> Bus Creator/6  "trajClear"
  Bus Selector2/1 -> MATLAB System/6
  MATLAB System/1 -> Bus Creator/1  "initQuat"
  MATLAB System/7 -> Bus Creator/7  "notDryRun"
  MATLAB System/4 -> Bus Creator/4  "navReset"
  Data Type Conversion/1 -> Bus Creator/5  "mode"
  MATLAB System/5 -> Data Type Conversion/1
  MATLAB System/3 -> Bus Creator/3  "simActivate"
  Bus Creator/1 -> rosCommands/1
  Delay/1 -> MATLAB System/12
  sensorOn/1 -> Delay/1
  MATLAB System/2 -> Bus Creator/2  "initPos"
  Bus Selector/1 -> MATLAB System/2
  Bus Selector3/1 -> MATLAB System/8
  proc_control set_mode/1 -> MATLAB System/1
  proc_control set_mode/2 -> Bus Selector/1
  proc_nav reset_pos/1 -> MATLAB System/3
  proc_nav reset_pos/2 -> Bus Selector1/1
  provider_rs485 kill_status/1 -> MATLAB System/5
  provider_rs485 kill_status/2 -> Bus Selector2/1
  proc_simulation start_simulation/1 -> MATLAB System/7
  proc_simulation start_simulation/2 -> Bus Selector3/1
  telemetry dryrun/1 -> MATLAB System/9
  telemetry dryrun/2 -> Bus Selector4/1
  proc_control reset_trajectory/1 -> MATLAB System/11
  proc_control reset_trajectory/2 -> Terminator/1

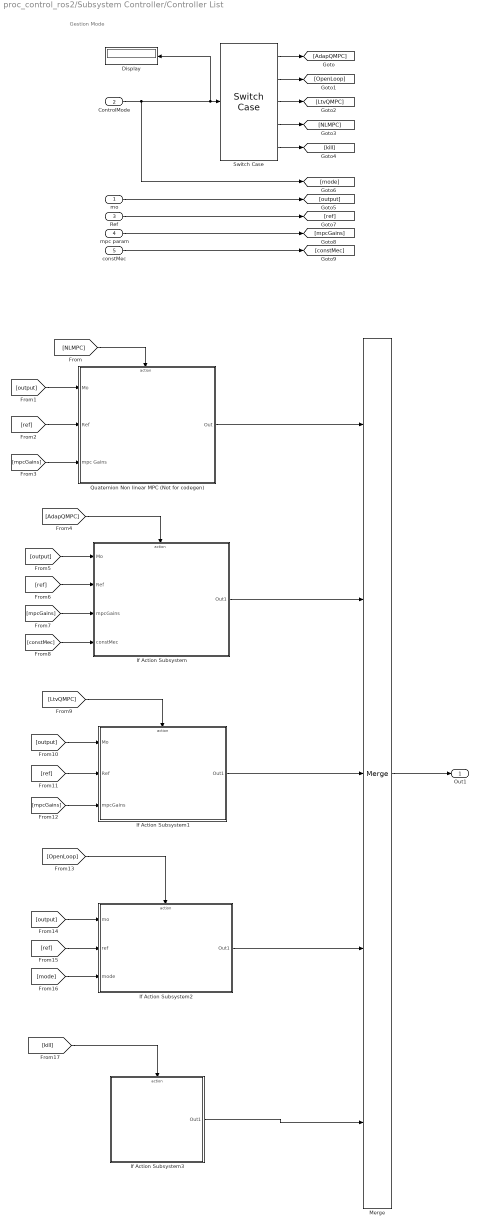
== system proc_control_ros2/Subsystem Controller/Controller List ==
  note: Gestion Mode
  mo : Inport
  ControlMode : Inport  Port=2  SampleTime=MPC.Ts
  Ref : Inport  Port=3
  mpc param : Inport  Port=4
  constMec : Inport  Port=5
  Display : Display
  If Action Subsystem : Subsystem  TreatAsAtomicUnit=on
  If Action Subsystem1 : Subsystem  TreatAsAtomicUnit=on
  If Action Subsystem2 : Subsystem  TreatAsAtomicUnit=on
  If Action Subsystem3 : Subsystem  TreatAsAtomicUnit=on
  Merge : Merge  Inputs=5
  Quaternion Non linear MPC (Not for codegen) : Subsystem  TreatAsAtomicUnit=on
  Switch Case : SwitchCase  CaseConditions="{ mode.control.adapQMpcMode,  mode.control.openLoopMode,    mode.control.LtvQMpcMode, mode.control.NlmpcMode}"
  Out1 : Outport
  wires:
  ControlMode/1 -> [mode], Display/1, Switch Case/1
  Switch Case/1 -> [AdapQMPC]
  Switch Case/2 -> [OpenLoop]
  Switch Case/3 -> [LtvQMPC]
  Switch Case/4 -> [NLMPC]
  Switch Case/5 -> [kill]
  mo/1 -> [output]
  Ref/1 -> [ref]
  mpc param/1 -> [mpcGains]
  constMec/1 -> [constMec]
  [NLMPC] -> Quaternion Non linear MPC (Not for codegen)/Action
  [output] -> Quaternion Non linear MPC (Not for codegen)/1(Mo)
  [ref] -> Quaternion Non linear MPC (Not for codegen)/2(Ref)
  [mpcGains] -> Quaternion Non linear MPC (Not for codegen)/3(mpc Gains)
  [AdapQMPC] -> If Action Subsystem/Action
  [output] -> If Action Subsystem/1(Mo)
  [mpcGains] -> If Action Subsystem/3(mpcGains)
  [ref] -> If Action Subsystem/2(Ref)
  [constMec] -> If Action Subsystem/4(constMec)
  If Action Subsystem/1(Out1) -> Merge/2
  Quaternion Non linear MPC (Not for codegen)/1(Out) -> Merge/1
  Merge/1 -> Out1/1
  [LtvQMPC] -> If Action Subsystem1/Action
  [output] -> If Action Subsystem1/1(Mo)
  [ref] -> If Action Subsystem1/2(Ref)
  [mpcGains] -> If Action Subsystem1/3(mpcGains)
  If Action Subsystem1/1(Out1) -> Merge/3
  [OpenLoop] -> If Action Subsystem2/Action
  [mode] -> If Action Subsystem2/3(mode)
  [output] -> If Action Subsystem2/1(mo)
  [ref] -> If Action Subsystem2/2(ref)
  If Action Subsystem2/1(Out1) -> Merge/4
  [kill] -> If Action Subsystem3/Action
  If Action Subsystem3/1(Out1) -> Merge/5
